simulink model "BoostConverter_iDesignMask"  (R2020b)
settings: Solver=FixedStepAuto  StartTime=0.0  StopTime=100  FixedStep=0.0015  RelTol=1e-3
libraries: PB_Library_Master x1, Lib_NM_JacobianCalc_TMATS x1, Lib_NM_NewtonRaphsonSolver_TMATS x1
settings Model: Creator=pmatt  LastModifiedBy=nbutler2
settings SFSimCC: CustomCodeUndefinedFunction=UseInterfaceOnly

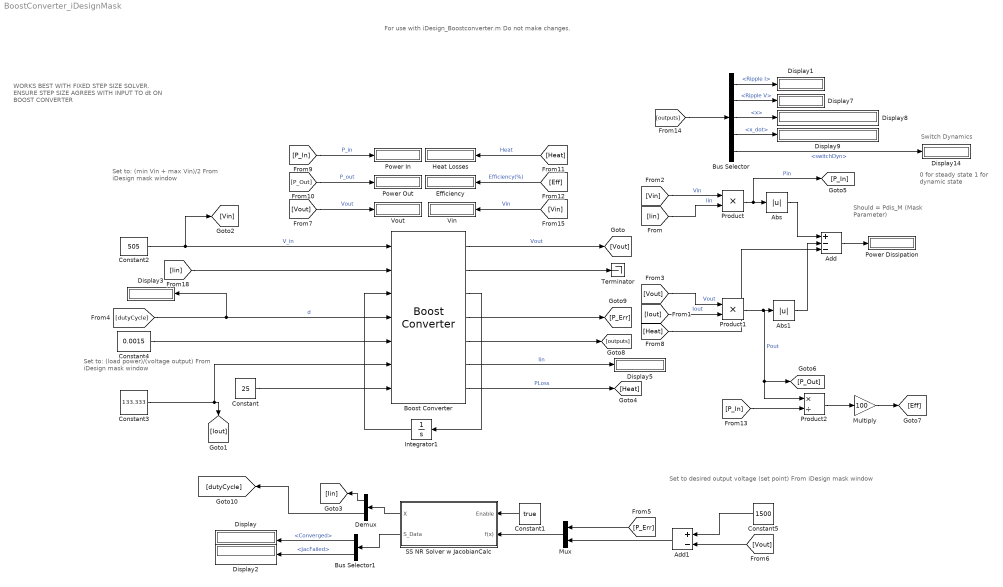
== system BoostConverter_iDesignMask ==
  note: WORKS BEST WITH FIXED
      | STEP SIZE SOLVER. ENSURE
      | STEP SIZE AGREES WITH INPUT
      | TO dt ON BOOST CONVERTER
  note: Set to:
      | (load power)/(voltage output)
      | From iDesign mask window
  note: Set to desired output voltage (set point)
      | From iDesign mask window
  note: Switch Dynamics
  note: Should = Pdis_M
      | (Mask Parameter)
  note: For use with iDesign_Boostconverter.m
      | Do not make changes.
  note: 0 for steady state
      | 1 for dynamic state
  note: Set to:
      | (min Vin + max Vin)/2
      | From iDesign mask window
  Abs : Abs
  Abs1 : Abs
  Add : Sum  Inputs=+--
  Add1 : Sum  Inputs=+-
  Boost Converter : PB_Library_Master/Boost Converter  Pdis_M=1  C_M=7.5e-08  L_M=0.00058366  Ron_M=0.036  RC_M=0.13302  RL_M=0.18419  QgTotal_M=8.4e-08  Vdiode_M=1.2  TRise_M=1.72e-07  TFall_M=7.8e-08  Fsw_M=250000  Vgate_M=4  n_MOSFET=1  MassEst_M=37.515  TempIn=Celsius  vOut=1500  pow=10000  minV=490  maxV=530  rippleMode=Use defaults (5% of voltage output and 10% of inductor current)  vRip=.05  iRip=.1  freqMode=Use default frequency (250 kHz)  freq=250e3
  Bus Selector : BusSelector  OutputSignals=Ripple I,Ripple V,x,x_dot,switchDyn
  Bus Selector1 : BusSelector  OutputSignals=Converged,JacFailed
  Constant : Constant  Value=25
  Constant1 : Constant  Value=true
  Constant2 : Constant  Value=505  VectorParams1D=off  SampleTime=-1
  Constant3 : Constant  Value=133.333
  Constant4 : Constant  Value=0.0015  VectorParams1D=off
  Constant5 : Constant  Value=1500
  Demux : Demux  Outputs=2
  Display{,1..3,5,7..9,14} (9 alike) : Display
      Display8 settings: Decimation=3
  Efficiency : Display
  Heat Losses : Display
  Integrator1 : Integrator  InitialCondition=[0;0]
  Multiply : Gain  Gain=100
  Mux : Mux  Inputs=2
  Power Dissipation : Display
  Power In : Display
  Power Out : Display
  Product : Product
  Product1 : Product
  Product2 : Product  Inputs=*/
  SS NR Solver w JacobianCalc : Subsystem  AncestorBlock=Lib_Solve_SSNRSolverJC_TMATS/SS NR Solver w JacobianCalc  mask(T-MATS: SS NR Solver w Jacobian Calc Library Block){SJac_Per_M=.01 * [1 -1; 1 -1], SNR_IC_M=[1;.5], SNR_DX_M=10, SNR_Mx_M=[100000;.99999], SNR_Mn_M=[0.00001;.0001], SJacobianAttempts_M=200, Cond_Limits_M=0.0001}
      mask prompts: SJac_Per_M "SJac_Per_M - Jacobian Perturbation size (frac)(nxm)"; SNR_IC_M "SNR_IC_M - Newton Raphson Initial Conditions (mx1)"; SNR_DX_M "SNR_DX_M - Newton Raphson step size limit (%) (1x1)"; SNR_Mx_M "SNR_Mx_M - Newton Raphson max limit (1x1 or mx1)"; SNR_Mn_M "SNR_Mn_M - Newton Raphson min limit (1x1 or mx1)"; SJacobianAttempts_M "SJacobianAttempts_M - Newton Raphson attempts before the Jacobian recalculation (1x1)"; Cond_Limits_M "Cond_Limits_M - Iteration Conditions Limits (mx1 or 1x1)"
      mask help:
      | The Steady State Newton Raphson Solver with Jacobian Calculator block will
      | supply the inputs to iteratively drive the outputs of a system to zero.
      |
      | This will be performed in three steps.
      | 1) Jabobian calculator sends Perturbations to the plant then calculates the plant
      | Jacboian based on the system response
      | 2) The Newton Raphson will use the inverse of the Jacobian to iteratively step the
      | system toward solution.
      | 3) Once the solution has satisfied the conditions the Newton Raphson is shut off.
      |
      | Simulation run time length should be selected as to give the Newton Raphson solver adequate time to develop a solution.
      mask init:
      | if isequal(size(SNR_Mx_M),size(SNR_IC_M))
      | elseif isequal(size(SNR_Mx_M),[1 1])
      | else
      |     disp('NR_Mx_Lim_M must be the same size as NR_IC_M or a constant')
      | end
      | 
      | if isequal(size(SNR_Mn_M),size(SNR_IC_M))
      | elseif isequal(size(SNR_Mn_M),[1 1])
      | else
      |     disp('NR_Mn_Lim_M must be the same size as NR_IC_M or a constant')
      | end
      mask Help: web(which('Solver_TMATS_SSNRwJC.html'),'-helpbrowser')
  Terminator : Terminator
  Vin : Display
  Vout : Display
  wires:
  [Iin] -> Boost Converter/2
  [Eff] -> Efficiency/1  "Efficiency(%)"
  Integrator1/1 -> Boost Converter/3
  Boost Converter/4 -> [P_Err]
  Boost Converter/5 -> [outputs]
  [Vout] -> Product1/1  "Vout"
  Constant2/1 -> Boost Converter/1, [Vin]  "V_in"
  Bus Selector/2 -> Display7/1  "<Ripple V>"
  Bus Selector/5 -> Display14/1  "<switchDyn>"
  Bus Selector/4 -> Display9/1  "<x_dot>"
  Boost Converter/7 -> [Heat]  "PLoss"
  [Iin] -> Product/2  "Iin"
  Boost Converter/6 -> Display5/1  "Iin"
  [Iout] -> Product1/2  "Iout"
  [P_Out] -> Power Out/1  "P_out"
  Abs1/1 -> Add/2
  Abs/1 -> Add/1
  [outputs] -> Bus Selector/1
  Bus Selector/1 -> Display1/1  "<Ripple I>"
  Boost Converter/3 -> Integrator1/1
  [Vin] -> Product/1  "Vin"
  [Heat] -> Heat Losses/1  "Heat"
  Bus Selector/3 -> Display8/1  "<x>"
  [P_In] -> Product2/2
  Add/1 -> Power Dissipation/1
  Product/1 -> [P_In], Abs/1  "Pin"
  Boost Converter/1 -> [Vout]  "Vout"
  Multiply/1 -> [Eff]
  Product2/1 -> Multiply/1
  [P_In] -> Power In/1  "P_in"
  Product1/1 -> [P_Out], Product2/1, Abs1/1  "Pout"
  Constant/1 -> Boost Converter/7
  Boost Converter/2 -> Terminator/1
  Constant3/1 -> Boost Converter/6, [Iout]
  [Heat] -> Add/3
  Constant4/1 -> Boost Converter/5
  [dutyCycle] -> Boost Converter/4, Display3/1  "d"
  Constant1/1 -> SS NR Solver w JacobianCalc/1(Enable)
  SS NR Solver w JacobianCalc/2(S_Data) -> Bus Selector1/1
  Bus Selector1/1 -> Display/1  "<Converged>"
  Bus Selector1/2 -> Display2/1  "<JacFailed>"
  [Vout] -> Add1/2
  Constant5/1 -> Add1/1
  Add1/1 -> Mux/2
  Mux/1 -> SS NR Solver w JacobianCalc/2(f(x))
  [P_Err] -> Mux/1
  SS NR Solver w JacobianCalc/1(X) -> Demux/1
  Demux/1 -> [Iin]
  Demux/2 -> [dutyCycle]
  [Vout] -> Vout/1  "Vout"
  [Vin] -> Vin/1  "Vin"

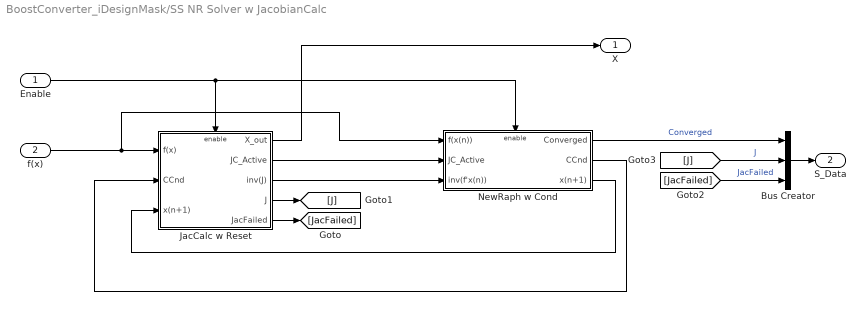
== system BoostConverter_iDesignMask/SS NR Solver w JacobianCalc ==
  Enable : Inport  PortDimensions=1
  f(x) : Inport  Port=2  PortDimensions=length(SNR_IC_M)
  Bus Creator : BusCreator  Inputs=3
  JacCalc w Reset : Subsystem  TreatAsAtomicUnit=on
  NewRaph w Cond : Subsystem  TreatAsAtomicUnit=on
  X : Outport  PortDimensions=length(SNR_IC_M)
  S_Data : Outport  Port=2  PortDimensions={1,[length(SNR_IC_M),length(SNR_IC_M)]}
  wires:
  JacCalc w Reset/1(X_out) -> X/1
  JacCalc w Reset/2(JC_Active) -> NewRaph w Cond/2(JC_Active)
  JacCalc w Reset/3(inv(J)) -> NewRaph w Cond/3(inv(f'x(n)))
  JacCalc w Reset/4(J) -> [J]
  NewRaph w Cond/2(CCnd) -> JacCalc w Reset/2(CCnd)
  f(x)/1 -> NewRaph w Cond/1(f(x(n))), JacCalc w Reset/1(f(x))
  NewRaph w Cond/3(x(n+1)) -> JacCalc w Reset/3(x(n+1))
  NewRaph w Cond/1(Converged) -> Bus Creator/1  "Converged"
  Enable/1 -> NewRaph w Cond/Enable, JacCalc w Reset/Enable
  JacCalc w Reset/5(JacFailed) -> [JacFailed]
  Bus Creator/1 -> S_Data/1
  [J] -> Bus Creator/2  "J"
  [JacFailed] -> Bus Creator/3  "JacFailed"

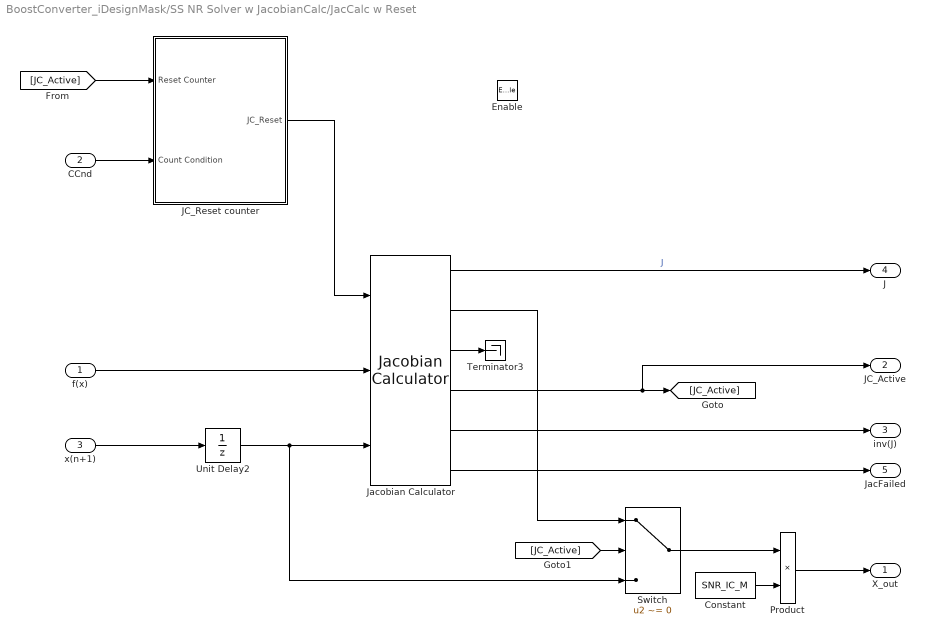
== system BoostConverter_iDesignMask/SS NR Solver w JacobianCalc/JacCalc w Reset ==
  f(x) : Inport  PortDimensions=length(SNR_IC_M)
  CCnd : Inport  Port=2  PortDimensions=1
  x(n+1) : Inport  Port=3  PortDimensions=length(SNR_IC_M)
  Enable : EnablePort
  Constant : Constant  Value=SNR_IC_M
  JC_Reset counter : Subsystem
  Jacobian Calculator : Lib_NM_JacobianCalc_TMATS/Jacobian Calculator  N_Per_M=SJac_Per_M
  Product : Product  RndMeth=Zero
  Switch : Switch  Criteria=u2 ~= 0  Threshold=1
  Terminator3 : Terminator
  Unit Delay2 : UnitDelay  InitialCondition=ones(length(SNR_IC_M),1)  SampleTime=-1  HasFrameUpgradeWarning=on
  X_out : Outport  PortDimensions=length(SNR_IC_M)
  JC_Active : Outport  Port=2  PortDimensions=1
  inv(J) : Outport  Port=3  PortDimensions=[length(SNR_IC_M),length(SNR_IC_M)]
  J : Outport  Port=4  PortDimensions=[length(SNR_IC_M),length(SNR_IC_M)]
  JacFailed : Outport  Port=5  PortDimensions=1
  wires:
  Jacobian Calculator/3 -> Terminator3/1
  Jacobian Calculator/2 -> Switch/1
  Jacobian Calculator/4 -> [JC_Active], JC_Active/1
  Unit Delay2/1 -> Switch/3, Jacobian Calculator/3
  Constant/1 -> Product/2
  Jacobian Calculator/5 -> inv(J)/1
  [JC_Active] -> JC_Reset counter/1(Reset Counter)
  Switch/1 -> Product/1
  Jacobian Calculator/1 -> J/1  "J"
  Product/1 -> X_out/1
  JC_Reset counter/1(JC_Reset) -> Jacobian Calculator/1
  x(n+1)/1 -> Unit Delay2/1
  CCnd/1 -> JC_Reset counter/2(Count Condition)
  [JC_Active] -> Switch/2
  f(x)/1 -> Jacobian Calculator/2
  Jacobian Calculator/6 -> JacFailed/1

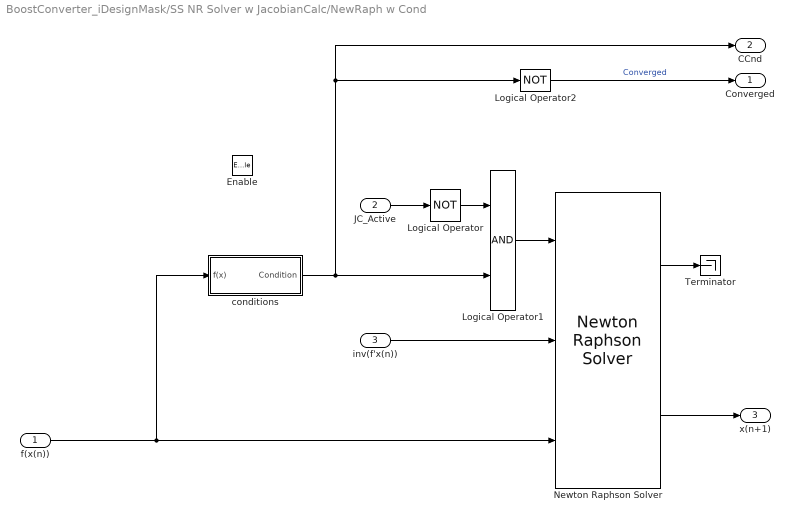
== system BoostConverter_iDesignMask/SS NR Solver w JacobianCalc/NewRaph w Cond ==
  f(x(n)) : Inport  PortDimensions=length(SNR_IC_M)
  JC_Active : Inport  Port=2  PortDimensions=1
  inv(f'x(n)) : Inport  Port=3  PortDimensions=[length(SNR_IC_M),length(SNR_IC_M)]
  Enable : EnablePort
  Logical Operator : Logic  Operator=NOT  AllPortsSameDT=off  OutDataTypeStr=boolean
  Logical Operator1 : Logic  AllPortsSameDT=off  OutDataTypeStr=boolean
  Logical Operator2 : Logic  Operator=NOT  AllPortsSameDT=off  OutDataTypeStr=boolean
  Newton Raphson Solver : Lib_NM_NewtonRaphsonSolver_TMATS/Newton Raphson Solver  NR_IC_M=ones(size(SNR_IC_M))  NR_dx_Lim_M=SNR_DX_M  NR_Mx_Lim_M=SNR_Mx_M./SNR_IC_M  NR_Mn_Lim_M=SNR_Mn_M./SNR_IC_M  BlkNm_M=double(gcb)
  Terminator : Terminator
  conditions : Subsystem
  Converged : Outport  PortDimensions={1,[length(SNR_IC_M),length(SNR_IC_M)]}
  CCnd : Outport  Port=2  PortDimensions=1
  x(n+1) : Outport  Port=3  PortDimensions=length(SNR_IC_M)
  wires:
  Logical Operator/1 -> Logical Operator1/1
  Logical Operator1/1 -> Newton Raphson Solver/1
  conditions/1(Condition) -> Logical Operator2/1, CCnd/1, Logical Operator1/2
  Logical Operator2/1 -> Converged/1  "Converged"
  JC_Active/1 -> Logical Operator/1
  inv(f'x(n))/1 -> Newton Raphson Solver/2
  Newton Raphson Solver/1 -> Terminator/1
  Newton Raphson Solver/2 -> x(n+1)/1
  f(x(n))/1 -> conditions/1(f(x)), Newton Raphson Solver/3

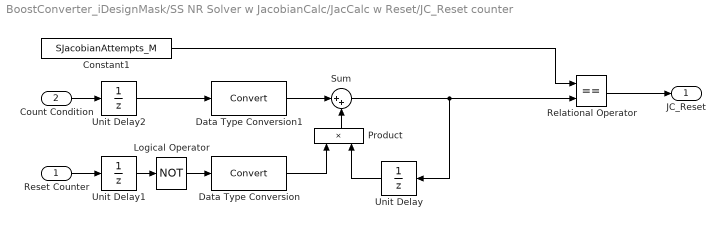
== system BoostConverter_iDesignMask/SS NR Solver w JacobianCalc/JacCalc w Reset/JC_Reset counter ==
  Reset Counter : Inport
  Count Condition : Inport  Port=2
  Constant1 : Constant  Value=SJacobianAttempts_M
  Data Type Conversion : DataTypeConversion
  Data Type Conversion1 : DataTypeConversion
  Logical Operator : Logic  Operator=NOT  AllPortsSameDT=off  OutDataTypeStr=boolean
  Product : Product  RndMeth=Zero
  Relational Operator : RelationalOperator  Operator===  OutDataTypeStr=boolean  RndMeth=Nearest
  Sum : Sum  Inputs=|++
  Unit Delay : UnitDelay  SampleTime=-1  HasFrameUpgradeWarning=on
  Unit Delay1 : UnitDelay  SampleTime=-1  HasFrameUpgradeWarning=on
  Unit Delay2 : UnitDelay  SampleTime=-1  HasFrameUpgradeWarning=on
  JC_Reset : Outport
  wires:
  Constant1/1 -> Relational Operator/1
  Relational Operator/1 -> JC_Reset/1
  Product/1 -> Sum/2
  Reset Counter/1 -> Unit Delay1/1
  Unit Delay/1 -> Product/2
  Data Type Conversion/1 -> Product/1
  Data Type Conversion1/1 -> Sum/1
  Unit Delay1/1 -> Logical Operator/1
  Logical Operator/1 -> Data Type Conversion/1
  Count Condition/1 -> Unit Delay2/1
  Unit Delay2/1 -> Data Type Conversion1/1
  Sum/1 -> Unit Delay/1, Relational Operator/2

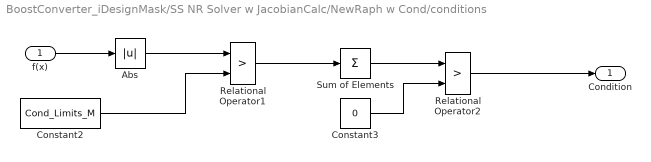
== system BoostConverter_iDesignMask/SS NR Solver w JacobianCalc/NewRaph w Cond/conditions ==
  f(x) : Inport
  Abs : Abs
  Constant2 : Constant  Value=Cond_Limits_M
  Constant3 : Constant  Value=0
  Relational Operator1 : RelationalOperator  Operator=>  OutDataTypeStr=boolean  RndMeth=Nearest
  Relational Operator2 : RelationalOperator  Operator=>  OutDataTypeStr=boolean  RndMeth=Nearest
  Sum of Elements : Sum  Inputs=+
  Condition : Outport
  wires:
  Constant2/1 -> Relational Operator1/2
  Relational Operator1/1 -> Sum of Elements/1
  Constant3/1 -> Relational Operator2/2
  Abs/1 -> Relational Operator1/1
  Sum of Elements/1 -> Relational Operator2/1
  f(x)/1 -> Abs/1
  Relational Operator2/1 -> Condition/1
